simulink model "Triggered_Subsystem_Ex"  (R2021b)
settings: Solver=VariableStepAuto  StartTime=0.0  StopTime=10.0  RelTol=1e-3
settings Model: Creator=t  LastModifiedBy=t

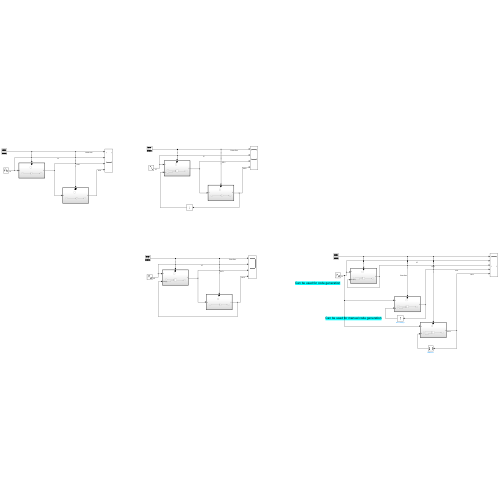
[thumbnail: Simulink's stored preview of the top-level diagram]
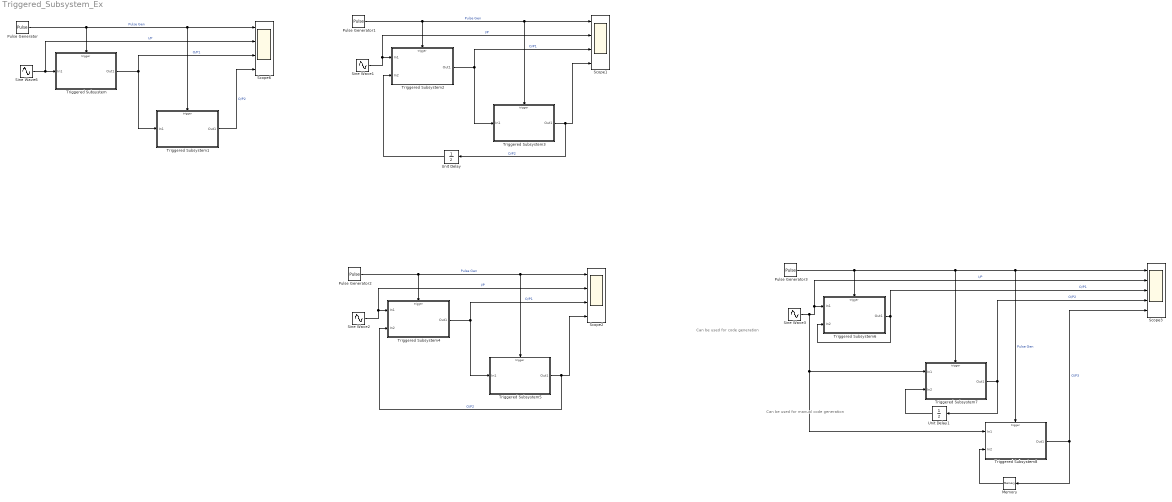
== system Triggered_Subsystem_Ex ==
  note: Can be used for code generation
  note: Can be used for manual code generation
  Memory : Memory
  Pulse Generator{,1..3} (4 alike) : DiscretePulseGenerator  Period=10  PulseWidth=5  SampleTime=0.2
  Scope1 : Scope  NumInputPorts=4
  Scope2 : Scope  NumInputPorts=4
  Scope3 : Scope  NumInputPorts=5
  Scope6 : Scope  NumInputPorts=4
  Sine Wave{1..3,6} (4 alike) : Sin  SampleTime=0.1
  Triggered Subsystem : Subsystem  TreatAsAtomicUnit=on
  Triggered Subsystem1 : Subsystem  TreatAsAtomicUnit=on
  Triggered Subsystem2 : Subsystem  TreatAsAtomicUnit=on
  Triggered Subsystem3 : Subsystem  TreatAsAtomicUnit=on
  Triggered Subsystem4 : Subsystem  TreatAsAtomicUnit=on
  Triggered Subsystem5 : Subsystem  TreatAsAtomicUnit=on
  Triggered Subsystem6 : Subsystem  TreatAsAtomicUnit=on
  Triggered Subsystem7 : Subsystem  TreatAsAtomicUnit=on
  Triggered Subsystem8 : Subsystem  TreatAsAtomicUnit=on
  Unit Delay : UnitDelay  SampleTime=-1  HasFrameUpgradeWarning=on
  Unit Delay1 : UnitDelay  SampleTime=-1  HasFrameUpgradeWarning=on
  wires:
  Sine Wave6/1 -> Scope6/2, Triggered Subsystem/1(In1)  "I/P"
  Pulse Generator/1 -> Triggered Subsystem/Trigger, Triggered Subsystem1/Trigger, Scope6/1  "Pulse Gen"
  Triggered Subsystem/1(Out1) -> Triggered Subsystem1/1(In1), Scope6/3  "O/P1"
  Triggered Subsystem1/1(Out1) -> Scope6/4  "O/P2"
  Triggered Subsystem3/1(Out1) -> Unit Delay/1, Scope1/4  "O/P2"
  Triggered Subsystem2/1(Out1) -> Scope1/3, Triggered Subsystem3/1(In1)  "O/P1"
  Pulse Generator1/1 -> Scope1/1, Triggered Subsystem3/Trigger, Triggered Subsystem2/Trigger  "Pulse Gen"
  Sine Wave1/1 -> Triggered Subsystem2/1(In1), Scope1/2  "I/P"
  Unit Delay/1 -> Triggered Subsystem2/2(In2)
  Sine Wave2/1 -> Scope2/2, Triggered Subsystem4/1(In1)  "I/P"
  Pulse Generator2/1 -> Triggered Subsystem4/Trigger, Triggered Subsystem5/Trigger, Scope2/1  "Pulse Gen"
  Triggered Subsystem4/1(Out1) -> Triggered Subsystem5/1(In1), Scope2/3  "O/P1"
  Triggered Subsystem5/1(Out1) -> Triggered Subsystem4/2(In2), Scope2/4  "O/P2"
  Triggered Subsystem7/1(Out1) -> Scope3/4, Unit Delay1/1  "O/P2"
  Triggered Subsystem6/1(Out1) -> Triggered Subsystem6/2(In2), Scope3/3  "O/P1"
  Pulse Generator3/1 -> Triggered Subsystem7/Trigger, Triggered Subsystem8/Trigger, Scope3/1, Triggered Subsystem6/Trigger  "Pulse Gen"
  Sine Wave3/1 -> Triggered Subsystem8/1(In1), Triggered Subsystem7/1(In1), Triggered Subsystem6/1(In1), Scope3/2  "I/P"
  Triggered Subsystem8/1(Out1) -> Memory/1, Scope3/5  "O/P3"
  Unit Delay1/1 -> Triggered Subsystem7/2(In2)
  Memory/1 -> Triggered Subsystem8/2(In2)

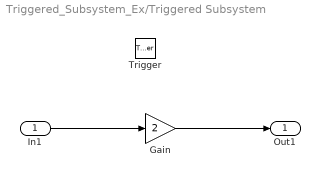
== system Triggered_Subsystem_Ex/Triggered Subsystem ==
  In1 : Inport
  Trigger : TriggerPort  VariantControl=(inherit)
  Gain : Gain  Gain=2
  Out1 : Outport
  wires:
  In1/1 -> Gain/1
  Gain/1 -> Out1/1

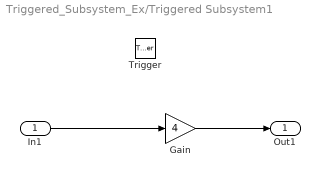
== system Triggered_Subsystem_Ex/Triggered Subsystem1 ==
  In1 : Inport
  Trigger : TriggerPort  VariantControl=(inherit)
  Gain : Gain  Gain=4
  Out1 : Outport
  wires:
  Gain/1 -> Out1/1
  In1/1 -> Gain/1

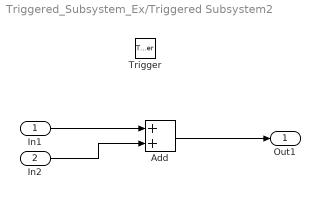
== system Triggered_Subsystem_Ex/Triggered Subsystem2 ==
  In1 : Inport
  In2 : Inport  Port=2
  Trigger : TriggerPort  VariantControl=(inherit)
  Add : Sum
  Out1 : Outport
  wires:
  Add/1 -> Out1/1
  In1/1 -> Add/1
  In2/1 -> Add/2

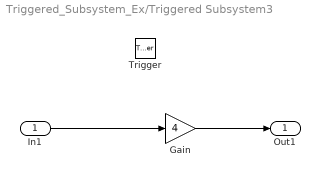
== system Triggered_Subsystem_Ex/Triggered Subsystem3 ==
  In1 : Inport
  Trigger : TriggerPort  VariantControl=(inherit)
  Gain : Gain  Gain=4
  Out1 : Outport
  wires:
  In1/1 -> Gain/1
  Gain/1 -> Out1/1

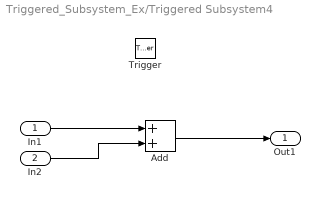
== system Triggered_Subsystem_Ex/Triggered Subsystem4 ==
  In1 : Inport
  In2 : Inport  Port=2  LatchByDelayingOutsideSignal=on
  Trigger : TriggerPort  VariantControl=(inherit)
  Add : Sum
  Out1 : Outport
  wires:
  In2/1 -> Add/2
  In1/1 -> Add/1
  Add/1 -> Out1/1

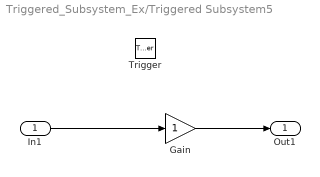
== system Triggered_Subsystem_Ex/Triggered Subsystem5 ==
  In1 : Inport
  Trigger : TriggerPort  VariantControl=(inherit)
  Gain : Gain
  Out1 : Outport
  wires:
  Gain/1 -> Out1/1
  In1/1 -> Gain/1

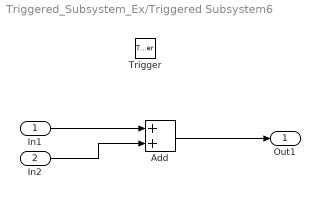
== system Triggered_Subsystem_Ex/Triggered Subsystem6 ==
  In1 : Inport
  In2 : Inport  Port=2  LatchByDelayingOutsideSignal=on
  Trigger : TriggerPort  VariantControl=(inherit)
  Add : Sum
  Out1 : Outport
  wires:
  Add/1 -> Out1/1
  In1/1 -> Add/1
  In2/1 -> Add/2

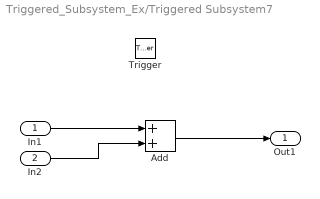
== system Triggered_Subsystem_Ex/Triggered Subsystem7 ==
  In1 : Inport
  In2 : Inport  Port=2
  Trigger : TriggerPort  VariantControl=(inherit)
  Add : Sum
  Out1 : Outport
  wires:
  In2/1 -> Add/2
  In1/1 -> Add/1
  Add/1 -> Out1/1

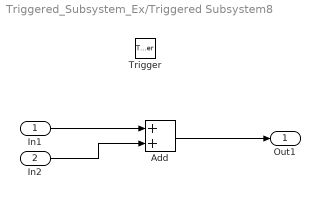
== system Triggered_Subsystem_Ex/Triggered Subsystem8 ==
  In1 : Inport
  In2 : Inport  Port=2
  Trigger : TriggerPort  VariantControl=(inherit)
  Add : Sum
  Out1 : Outport
  wires:
  Add/1 -> Out1/1
  In1/1 -> Add/1
  In2/1 -> Add/2
